simulink model "filecuaho"  (R2016b)
settings: Solver=VariableStepAuto  StartTime=0.0  StopTime=10.0  RelTol=1e-3
undefined symbols (not defined in the file): KACC_ACCT_CLR_NIDL_INIT, KACC_ACCUT_STATE_A, KACC_ACCUT_STATE_B, KACC_ACCUT_SW, KACC_ACTQSW, KACC_CLD, KACC_CLD_REQ_HYS, KACC_CLD_REQ_SW, KACC_COLPD, KACC_COMP_INRT, KACC_COMPTYPE_FIXED, KACC_COMPTYPE_VAR, KACC_CTTM_ACE, KACC_CTTM_ACON, KACC_CTTM_CRK, KACC_CTTM_FAN, KACC_CTTM_GRD, KACC_CTTM_IRS, KACC_CTTM_NAC, KACC_DIFFEVATEMPMAX, KACC_DIFFEVATEMPMIN, KACC_EVAT_ELSE, KACC_EVAT_ELSE_SW, KACC_EVATMPCUT_SW, KACC_EVATUPL_ELSE, KACC_EVATUPL_ELSE_SW, KACC_FANREQ_SW, KACC_FORCEDACON, KACC_HCAPS, KACC_HCAPS_HYS, KACC_HCCTTM, KACC_HCGRA, KACC_HCGRA_HYS, KACC_HCRGR, KACC_HCVS1, KACC_HCVS1_HYS, KACC_HCVS2, KACC_HCVS2_HYS, KACC_HEATUP_CE, KACC_HEATUP_CE_HYS, KACC_HEATUP_DRV2IDL, KACC_HEATUP_IDL2DRV, KACC_HEATUP_NE, KACC_HEATUP_NE_HYS, KACC_HIPS_ACOF, KACC_HIPS_ACON, KACC_LOPS_ACOF, KACC_LOPS_ACON, KACC_LYR3TR_ACHLD, KACC_NEW_RPM, KACC_OFDL_SW, KACC_OFDL_VCV, KACC_ONDL_SW, KACC_RECCP, KACC_RECCP_HYS, KACC_RECDLY, KACC_RECVS, KACC_S1_THWMAX, KACC_S1TM_THWULMT, KACC_SHLT_2CYL ... (+137)
libraries: lib2011b x727, SUBSYSTEM_LIB_CNV x30, SUBSYSTEM_LIB_ESC x2, SUBSYSTEM_LIB_AUX x1
(part 5 of 5)

== system filecuaho/acc_xaccuton/acc_accutreq/cal_cuttime ==
  note: 加速要求エアコンカットフラグ
  note: エアコンカット要求前にvcvcut要求があった場合は、
      | vcvcutを実行した時間だけエアコンカット維持時間をoffsetする
  xlacni : Inport
  xlacfs : Inport  Port=2
  xlacfs_iss : Inport  Port=3
  w_vcv_cut_time : Inport  Port=4
  xacct1 : Inport  Port=5
  xacct4 : Inport  Port=6
  xacuthil : Inport  Port=7
  xactempcut : Inport  Port=8
  MC_Add3 : lib2011b/Simulink Original/Math Operations/MC_Add  Inputs=+-  CollapseDim=1  SampleTime=-1  InputSameDT=on  OutMin=[]  OutMax=[]  OutDataTypeStr=single
  MC_Constant : lib2011b/Simulink Original/Sources/MC_Constant  Value=KACC_CTTM_NAC  datatype=Inherit: Inherit from 'Constant value'  SampleTime=inf  FramePeriod=inf  OutMin=[]  OutMax=[]  OutDataTypeStr=Inherit: Inherit from 'Constant value'
  MC_Constant1 : lib2011b/Simulink Original/Sources/MC_Constant  Value=KACC_CTTM_CRK  datatype=Inherit: Inherit from 'Constant value'  SampleTime=inf  FramePeriod=inf  OutMin=[]  OutMax=[]  OutDataTypeStr=Inherit: Inherit from 'Constant value'
  MC_Constant4 : lib2011b/Simulink Original/Sources/MC_Constant  Value=KACC_CTTM_IRS  datatype=Inherit: Inherit from 'Constant value'  SampleTime=inf  FramePeriod=inf  OutMin=[]  OutMax=[]  OutDataTypeStr=Inherit: Inherit from 'Constant value'
  MC_Constant5 : lib2011b/Simulink Original/Sources/MC_Constant  Value=KACC_CTTM_GRD  datatype=Inherit: Inherit from 'Constant value'  SampleTime=inf  FramePeriod=inf  OutMin=[]  OutMax=[]  OutDataTypeStr=Inherit: Inherit from 'Constant value'
  MC_Constant{6..9} (4 alike) : lib2011b/Simulink Original/Sources/MC_Constant  Value=0  datatype=single  SampleTime=inf  FramePeriod=inf  OutMin=[]  OutMax=[]  OutDataTypeStr=single
  MC_Edge2 : lib2011b/Mazda Library/Other/MC_Edge
  MC_LogicalOperator : lib2011b/Simulink Original/Logic and Bit Operations/MC_LogicalOperator  SelectedOperator=NOT  Inputs=2  SampleTime=-1  AllPortsSameDT=off  OutDataTypeStr=boolean
  MC_LogicalOperator1 : lib2011b/Simulink Original/Logic and Bit Operations/MC_LogicalOperator  SelectedOperator=OR  Inputs=3  SampleTime=-1  AllPortsSameDT=off  OutDataTypeStr=boolean
  MC_LogicalOperator3 : lib2011b/Simulink Original/Logic and Bit Operations/MC_LogicalOperator  SelectedOperator=OR  Inputs=4  SampleTime=-1  AllPortsSameDT=off  OutDataTypeStr=boolean
  MC_MinMax : lib2011b/Simulink Original/Math Operations/MC_MinMax  Function=max  Inputs=4  SampleTime=-1  InputSameDT=on  OutMin=[]  OutMax=[]
  MC_Switch{1,3..4,6} (4 alike) : lib2011b/Simulink Original/Signal Routing/MC_Switch  Criteria=u2 ~= 0  Threshold=0  SampleTime=-1  InputSameDT=on  OutMin=[]  OutMax=[]  AllowDiffInputSizes=off
  MC_UnitDelay1 : lib2011b/Simulink Original/Discrete/MC_UnitDelay  InitialCondition=0  InputProcessing=Inherited  SampleTime=-1  StateName=delay_yclcn_b20m9498
      settings: StateMustResolveToSignalObject=off  StateStorageClass=ExportedGlobal
  Switch5 : lib2011b/Simulink Original/Signal Routing/MC_Switch  Criteria=u2 ~= 0  Threshold=0  SampleTime=-1  InputSameDT=on  OutMin=[]  OutMax=[]  AllowDiffInputSizes=off
  xaccut_wicnt : Outport
  accut_reqtime : Outport  Port=2
  wires:
  MC_Constant/1 -> MC_Switch4/1
  MC_Constant1/1 -> MC_Switch1/1
  MC_Constant4/1 -> MC_Switch3/1
  [xlacfs] -> MC_Switch1/2
  xlacni/1 -> [xlacni]
  xlacfs/1 -> [xlacfs]
  xlacfs_iss/1 -> [xlacfs_iss]
  [xlacni] -> MC_Switch4/2
  [xlacfs_iss] -> MC_Switch3/2
  MC_MinMax/1 -> MC_Add3/1  "accut_reqtime_pre"
  [xlacni] -> MC_LogicalOperator1/1
  [xlacfs] -> MC_LogicalOperator1/2
  [xlacfs_iss] -> MC_LogicalOperator1/3
  MC_LogicalOperator1/1 -> xaccut_wicnt/1, MC_LogicalOperator/1  "xaccut_wicnt"
  MC_Constant5/1 -> MC_Switch6/1
  MC_Constant6/1 -> MC_Switch6/3
  MC_Constant8/1 -> MC_Switch1/3
  MC_Constant9/1 -> MC_Switch3/3
  MC_LogicalOperator/1 -> MC_Switch6/2
  MC_Constant7/1 -> MC_Switch4/3
  MC_Switch6/1 -> MC_MinMax/1
  MC_Switch4/1 -> MC_MinMax/2
  MC_Switch1/1 -> MC_MinMax/3
  MC_Switch3/1 -> MC_MinMax/4
  w_vcv_cut_time/1 -> [w_vcv_cut_time]  "w_vcv_cut_time"
  xacct1/1 -> [xacct1]
  xacct4/1 -> [xacct4]
  xacuthil/1 -> [xacuthil]
  xactempcut/1 -> [xactempcut]
  MC_Edge2/1 -> Switch5/2
  Switch5/1 -> MC_UnitDelay1/1, MC_Add3/2
  MC_UnitDelay1/1 -> Switch5/3
  [w_vcv_cut_time] -> Switch5/1
  MC_LogicalOperator3/1 -> MC_Edge2/1
  [xacct1] -> MC_LogicalOperator3/1
  [xacct4] -> MC_LogicalOperator3/2
  [xacuthil] -> MC_LogicalOperator3/3
  [xactempcut] -> MC_LogicalOperator3/4
  MC_Add3/1 -> accut_reqtime/1  "accut_reqtime"

== system filecuaho/acc_xaccuton/acc_accutreq/do_xacct1 ==
  xrload : Inport
  apsfil : Inport  Port=2
  gearp : Inport  Port=3
  w_tsmpl : Inport  Port=4
  Constant1 : lib2011b/Simulink Original/Sources/MC_Constant  Value=KSAVAC  datatype=Inherit: Inherit from 'Constant value'  SampleTime=inf  FramePeriod=inf  OutMin=[]  OutMax=[]  OutDataTypeStr=Inherit: Inherit from 'Constant value'
  Constant11 : lib2011b/Simulink Original/Sources/MC_Constant  Value=KSAVAC_HYS  datatype=Inherit: Inherit from 'Constant value'  SampleTime=inf  FramePeriod=inf  OutMin=[]  OutMax=[]  OutDataTypeStr=Inherit: Inherit from 'Constant value'
  LogicalOperator10 : lib2011b/Simulink Original/Logic and Bit Operations/MC_LogicalOperator  SelectedOperator=AND  Inputs=2  SampleTime=-1  AllPortsSameDT=off  OutDataTypeStr=boolean
  MC_Constant1 : lib2011b/Simulink Original/Sources/MC_Constant  Value=true  datatype=Inherit: Inherit from 'Constant value'  SampleTime=inf  FramePeriod=inf  OutMin=[]  OutMax=[]  OutDataTypeStr=Inherit: Inherit from 'Constant value'
  MC_Constant5 : lib2011b/Simulink Original/Sources/MC_Constant  Value=false  datatype=Inherit: Inherit from 'Constant value'  SampleTime=inf  FramePeriod=inf  OutMin=[]  OutMax=[]  OutDataTypeStr=Inherit: Inherit from 'Constant value'
  MC_Constant7 : lib2011b/Simulink Original/Sources/MC_Constant  Value=0  datatype=single  SampleTime=inf  FramePeriod=inf  OutMin=[]  OutMax=[]  OutDataTypeStr=single
  MC_DownCountTimer : lib2011b/Mazda Library/Timer/MC_DownCountTimer
      settings: AttributesFormatString=DownCountTimer
  MC_Edge : SUBSYSTEM_LIB_CNV/RiseEdge
      settings: AttributesFormatString=RISE
  MC_Hysteresis4 : SUBSYSTEM_LIB_CNV/TrueHys
      settings: AttributesFormatString=True
  MC_LogicalOperator : lib2011b/Simulink Original/Logic and Bit Operations/MC_LogicalOperator  SelectedOperator=NOT  Inputs=2  SampleTime=-1  AllPortsSameDT=off  OutDataTypeStr=boolean
  MC_RelationalOperator3 : lib2011b/Simulink Original/Logic and Bit Operations/MC_RelationalOperator  Operator=>  SampleTime=-1  InputSameDT=on  OutDataTypeStr=boolean
  MC_Table : lib2011b/Simulink Original/Lookup Tables/MC_Table_i  Label=TACC_TLACT  InputValues=TACC_TLACT_X  calsw_x=off  OutputValues=TACC_TLACT_Y  LsbValue=LSB_TACC_TLACT_Y  OffsetValue=OFFSET_TACC_TLACT_Y
      settings: AttributesFormatString=%<Label>\nX-axis %<calsw_x>
  xacct1 : Outport
  wires:
  apsfil/1 -> MC_Hysteresis4/1
  xrload/1 -> LogicalOperator10/1
  MC_Hysteresis4/1 -> LogicalOperator10/2  "xavact"
  Constant11/1 -> MC_Hysteresis4/3
  Constant1/1 -> MC_Hysteresis4/2
  MC_Constant5/1 -> MC_Edge/2
  LogicalOperator10/1 -> MC_Edge/1, MC_LogicalOperator/1
  MC_Constant1/1 -> MC_DownCountTimer/3
  MC_LogicalOperator/1 -> MC_DownCountTimer/1
  MC_Constant7/1 -> MC_RelationalOperator3/2
  MC_DownCountTimer/1 -> MC_RelationalOperator3/1  "tacct1"
  MC_RelationalOperator3/1 -> xacct1/1  "xacct1"
  w_tsmpl/1 -> MC_DownCountTimer/5
  gearp/1 -> MC_Table/1
  MC_Table/1 -> MC_DownCountTimer/4
  MC_Edge/1 -> MC_DownCountTimer/2  "xacct1_req"

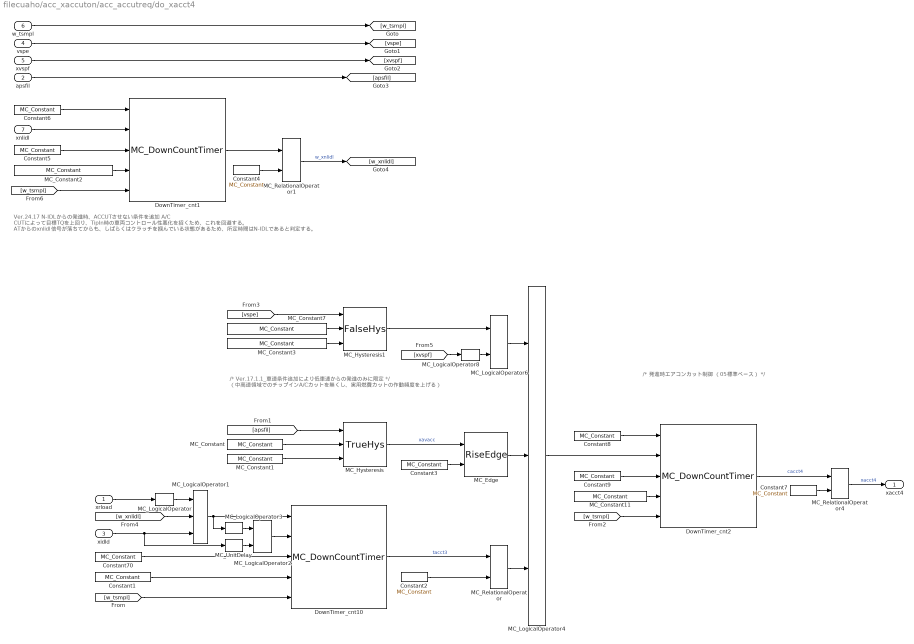
== system filecuaho/acc_xaccuton/acc_accutreq/do_xacct4 ==
  note: /* 発進時エアコンカット制御 （05標準ベース） */
  note: /* Ver.17.1.1_車速条件追加により低車速からの発進のみに限定 */
      |
      | （中高速領域でのチップインA/Cカットを無くし、実用燃費カットの作動頻度を上げる）
  note: Ver.24.17 N-IDLからの発進時、ACCUTさせない条件を追加
      | A/C CUTによって目標TQを上回り、TipIn時の車両コントロール性悪化を招くため、これを回避する。
      | ATからのxnlidl信号が落ちてからも、しばらくはクラッチを掴んでいる状態があるため、所定時間はN-IDLであると判定する。
  xrload : Inport
  apsfil : Inport  Port=2
  xidld : Inport  Port=3
  vspe : Inport  Port=4
  xvspf : Inport  Port=5
  w_tsmpl : Inport  Port=6
  xnlidl : Inport  Port=7
  Constant1 : lib2011b/Simulink Original/Sources/MC_Constant  Value=KLACT3  datatype=Inherit: Inherit from 'Constant value'  SampleTime=inf  FramePeriod=inf  OutMin=[]  OutMax=[]  OutDataTypeStr=Inherit: Inherit from 'Constant value'
  Constant2 : lib2011b/Simulink Original/Sources/MC_Constant  Value=0  datatype=single  SampleTime=inf  FramePeriod=inf  OutMin=[]  OutMax=[]  OutDataTypeStr=single
  Constant3 : lib2011b/Simulink Original/Sources/MC_Constant  Value=false  datatype=Inherit: Inherit from 'Constant value'  SampleTime=inf  FramePeriod=inf  OutMin=[]  OutMax=[]  OutDataTypeStr=Inherit: Inherit from 'Constant value'
  Constant4 : lib2011b/Simulink Original/Sources/MC_Constant  Value=0  datatype=single  SampleTime=inf  FramePeriod=inf  OutMin=[]  OutMax=[]  OutDataTypeStr=single
  Constant5 : lib2011b/Simulink Original/Sources/MC_Constant  Value=true  datatype=Inherit: Inherit from 'Constant value'  SampleTime=inf  FramePeriod=inf  OutMin=[]  OutMax=[]  OutDataTypeStr=Inherit: Inherit from 'Constant value'
  Constant6 : lib2011b/Simulink Original/Sources/MC_Constant  Value=false  datatype=Inherit: Inherit from 'Constant value'  SampleTime=inf  FramePeriod=inf  OutMin=[]  OutMax=[]  OutDataTypeStr=Inherit: Inherit from 'Constant value'
  Constant7 : lib2011b/Simulink Original/Sources/MC_Constant  Value=0  datatype=single  SampleTime=inf  FramePeriod=inf  OutMin=[]  OutMax=[]  OutDataTypeStr=single
  Constant70 : lib2011b/Simulink Original/Sources/MC_Constant  Value=true  datatype=Inherit: Inherit from 'Constant value'  SampleTime=inf  FramePeriod=inf  OutMin=[]  OutMax=[]  OutDataTypeStr=Inherit: Inherit from 'Constant value'
  Constant8 : lib2011b/Simulink Original/Sources/MC_Constant  Value=false  datatype=Inherit: Inherit from 'Constant value'  SampleTime=inf  FramePeriod=inf  OutMin=[]  OutMax=[]  OutDataTypeStr=Inherit: Inherit from 'Constant value'
  Constant9 : lib2011b/Simulink Original/Sources/MC_Constant  Value=true  datatype=Inherit: Inherit from 'Constant value'  SampleTime=inf  FramePeriod=inf  OutMin=[]  OutMax=[]  OutDataTypeStr=Inherit: Inherit from 'Constant value'
  DownTimer_cnt1 : lib2011b/Mazda Library/Timer/MC_DownCountTimer
      settings: AttributesFormatString=DownCountTimer
  DownTimer_cnt10 : lib2011b/Mazda Library/Timer/MC_DownCountTimer
      settings: AttributesFormatString=DownCountTimer
  DownTimer_cnt2 : lib2011b/Mazda Library/Timer/MC_DownCountTimer
      settings: AttributesFormatString=DownCountTimer
  MC_Constant : lib2011b/Simulink Original/Sources/MC_Constant  Value=KSAVCC  datatype=Inherit: Inherit from 'Constant value'  SampleTime=inf  FramePeriod=inf  OutMin=[]  OutMax=[]  OutDataTypeStr=Inherit: Inherit from 'Constant value'
  MC_Constant1 : lib2011b/Simulink Original/Sources/MC_Constant  Value=KSAVCC_HYS  datatype=Inherit: Inherit from 'Constant value'  SampleTime=inf  FramePeriod=inf  OutMin=[]  OutMax=[]  OutDataTypeStr=Inherit: Inherit from 'Constant value'
  MC_Constant11 : lib2011b/Simulink Original/Sources/MC_Constant  Value=KACC_CTTM_ACE  datatype=Inherit: Inherit from 'Constant value'  SampleTime=inf  FramePeriod=inf  OutMin=[]  OutMax=[]  OutDataTypeStr=Inherit: Inherit from 'Constant value'
  MC_Constant2 : lib2011b/Simulink Original/Sources/MC_Constant  Value=KACC_ACCT_CLR_NIDL_INIT  datatype=Inherit: Inherit from 'Constant value'  SampleTime=inf  FramePeriod=inf  OutMin=[]  OutMax=[]  OutDataTypeStr=Inherit: Inherit from 'Constant value'
  MC_Constant3 : lib2011b/Simulink Original/Sources/MC_Constant  Value=KACC_START_VSP_HYS  datatype=Inherit: Inherit from 'Constant value'  SampleTime=inf  FramePeriod=inf  OutMin=[]  OutMax=[]  OutDataTypeStr=Inherit: Inherit from 'Constant value'
  MC_Constant7 : lib2011b/Simulink Original/Sources/MC_Constant  Value=KACC_START_VSP  datatype=Inherit: Inherit from 'Constant value'  SampleTime=inf  FramePeriod=inf  OutMin=[]  OutMax=[]  OutDataTypeStr=Inherit: Inherit from 'Constant value'
  MC_Edge : SUBSYSTEM_LIB_CNV/RiseEdge
      settings: AttributesFormatString=RISE
  MC_Hysteresis : SUBSYSTEM_LIB_CNV/TrueHys
      settings: AttributesFormatString=True
  MC_Hysteresis1 : SUBSYSTEM_LIB_CNV/FalseHys
      settings: AttributesFormatString=False
  MC_LogicalOperator : lib2011b/Simulink Original/Logic and Bit Operations/MC_LogicalOperator  SelectedOperator=NOT  Inputs=2  SampleTime=-1  AllPortsSameDT=off  OutDataTypeStr=boolean
  MC_LogicalOperator1 : lib2011b/Simulink Original/Logic and Bit Operations/MC_LogicalOperator  SelectedOperator=OR  Inputs=3  SampleTime=-1  AllPortsSameDT=off  OutDataTypeStr=boolean
  MC_LogicalOperator2 : lib2011b/Simulink Original/Logic and Bit Operations/MC_LogicalOperator  SelectedOperator=AND  Inputs=2  SampleTime=-1  AllPortsSameDT=off  OutDataTypeStr=boolean
  MC_LogicalOperator3 : lib2011b/Simulink Original/Logic and Bit Operations/MC_LogicalOperator  SelectedOperator=NOT  Inputs=2  SampleTime=-1  AllPortsSameDT=off  OutDataTypeStr=boolean
  MC_LogicalOperator4 : lib2011b/Simulink Original/Logic and Bit Operations/MC_LogicalOperator  SelectedOperator=AND  Inputs=3  SampleTime=-1  AllPortsSameDT=off  OutDataTypeStr=boolean
  MC_LogicalOperator6 : lib2011b/Simulink Original/Logic and Bit Operations/MC_LogicalOperator  SelectedOperator=AND  Inputs=2  SampleTime=-1  AllPortsSameDT=off  OutDataTypeStr=boolean
  MC_LogicalOperator8 : lib2011b/Simulink Original/Logic and Bit Operations/MC_LogicalOperator  SelectedOperator=NOT  Inputs=2  SampleTime=-1  AllPortsSameDT=off  OutDataTypeStr=boolean
  MC_RelationalOperator : lib2011b/Simulink Original/Logic and Bit Operations/MC_RelationalOperator  Operator=>  SampleTime=-1  InputSameDT=on  OutDataTypeStr=boolean
  MC_RelationalOperator1 : lib2011b/Simulink Original/Logic and Bit Operations/MC_RelationalOperator  Operator=>  SampleTime=-1  InputSameDT=on  OutDataTypeStr=boolean
  MC_RelationalOperator4 : lib2011b/Simulink Original/Logic and Bit Operations/MC_RelationalOperator  Operator=>  SampleTime=-1  InputSameDT=on  OutDataTypeStr=boolean
  MC_UnitDelay : lib2011b/Simulink Original/Discrete/MC_UnitDelay  InitialCondition=0  InputProcessing=Inherited  SampleTime=-1  StateName=delay_yclcn_b20m9499
      settings: StateMustResolveToSignalObject=off  StateStorageClass=ExportedGlobal
  xacct4 : Outport
  wires:
  MC_Constant1/1 -> MC_Hysteresis/3
  MC_Constant/1 -> MC_Hysteresis/2
  MC_LogicalOperator2/1 -> DownTimer_cnt10/2
  MC_UnitDelay/1 -> MC_LogicalOperator2/2
  MC_LogicalOperator3/1 -> MC_LogicalOperator2/1
  xidld/1 -> MC_UnitDelay/1, MC_LogicalOperator1/3
  MC_LogicalOperator/1 -> MC_LogicalOperator1/1
  MC_LogicalOperator1/1 -> DownTimer_cnt10/1, MC_LogicalOperator3/1
  xrload/1 -> MC_LogicalOperator/1
  Constant1/1 -> DownTimer_cnt10/4
  Constant70/1 -> DownTimer_cnt10/3
  Constant3/1 -> MC_Edge/2
  Constant2/1 -> MC_RelationalOperator/2
  DownTimer_cnt10/1 -> MC_RelationalOperator/1  "tacct3"
  MC_Hysteresis/1 -> MC_Edge/1  "xavacc"
  w_tsmpl/1 -> [w_tsmpl]
  [w_tsmpl] -> DownTimer_cnt10/5
  MC_RelationalOperator/1 -> MC_LogicalOperator4/3
  MC_LogicalOperator4/1 -> DownTimer_cnt2/2
  [w_tsmpl] -> DownTimer_cnt2/5
  Constant8/1 -> DownTimer_cnt2/1
  Constant9/1 -> DownTimer_cnt2/3
  MC_RelationalOperator4/1 -> xacct4/1  "xacct4"
  DownTimer_cnt2/1 -> MC_RelationalOperator4/1  "cacct4"
  vspe/1 -> [vspe]
  xvspf/1 -> [xvspf]
  [xvspf] -> MC_LogicalOperator8/1
  MC_Constant11/1 -> DownTimer_cnt2/4
  Constant7/1 -> MC_RelationalOperator4/2
  MC_Edge/1 -> MC_LogicalOperator4/2
  MC_LogicalOperator6/1 -> MC_LogicalOperator4/1
  MC_LogicalOperator8/1 -> MC_LogicalOperator6/2
  MC_Hysteresis1/1 -> MC_LogicalOperator6/1
  [vspe] -> MC_Hysteresis1/1
  MC_Constant7/1 -> MC_Hysteresis1/2
  MC_Constant3/1 -> MC_Hysteresis1/3
  apsfil/1 -> [apsfil]
  [apsfil] -> MC_Hysteresis/1
  xnlidl/1 -> DownTimer_cnt1/2
  [w_xnlidl] -> MC_LogicalOperator1/2
  Constant4/1 -> MC_RelationalOperator1/2
  DownTimer_cnt1/1 -> MC_RelationalOperator1/1
  MC_RelationalOperator1/1 -> [w_xnlidl]  "w_xnlidl"
  Constant5/1 -> DownTimer_cnt1/3
  Constant6/1 -> DownTimer_cnt1/1
  [w_tsmpl] -> DownTimer_cnt1/5
  MC_Constant2/1 -> DownTimer_cnt1/4

== system filecuaho/acc_xaccuton/acc_accutreq/do_xacflostcut ==
  xcol : Inport
  evatemp : Inport  Port=2
  Constant14 : lib2011b/Simulink Original/Sources/MC_Constant  Value=KACC_VCD_EVATMP_HYS  datatype=Inherit: Inherit from 'Constant value'  SampleTime=inf  FramePeriod=inf  OutMin=[]  OutMax=[]  OutDataTypeStr=Inherit: Inherit from 'Constant value'
  Constant5 : lib2011b/Simulink Original/Sources/MC_Constant  Value=KACC_VCD_EVATMP  datatype=Inherit: Inherit from 'Constant value'  SampleTime=inf  FramePeriod=inf  OutMin=[]  OutMax=[]  OutDataTypeStr=Inherit: Inherit from 'Constant value'
  MC_Add : lib2011b/Simulink Original/Math Operations/MC_Add  Inputs=++  CollapseDim=1  SampleTime=-1  OutMin=[]  OutMax=[]  OutDataTypeStr=single
  MC_Hysteresis : lib2011b/Mazda Library/Other/MC_Hysteresis  outtype=False
      settings: AttributesFormatString=%<outtype>
  MC_LogicalOperator4 : lib2011b/Simulink Original/Logic and Bit Operations/MC_LogicalOperator  SelectedOperator=AND  Inputs=2  SampleTime=-1  AllPortsSameDT=off  OutDataTypeStr=boolean
  MC_LogicalOperator5 : lib2011b/Simulink Original/Logic and Bit Operations/MC_LogicalOperator  SelectedOperator=NOT  Inputs=2  SampleTime=-1  AllPortsSameDT=off  OutDataTypeStr=boolean
  xacflostcut : Outport
  wires:
  xcol/1 -> MC_LogicalOperator5/1
  MC_LogicalOperator5/1 -> MC_LogicalOperator4/1
  Constant5/1 -> MC_Hysteresis/3, MC_Add/2
  Constant14/1 -> MC_Add/1
  MC_Add/1 -> MC_Hysteresis/2
  evatemp/1 -> MC_Hysteresis/1
  MC_Hysteresis/1 -> MC_LogicalOperator4/2
  MC_LogicalOperator4/1 -> xacflostcut/1  "xacflostcut"

== system filecuaho/acc_xaccuton/acc_accutreq/do_xacfrpm ==
  ne : Inport
  xclcn : Inport  Port=2
  xaltcalflg : Inport  Port=3
  MC_Add : lib2011b/Simulink Original/Math Operations/MC_Add  Inputs=-+  CollapseDim=1  SampleTime=-1  InputSameDT=on  OutMin=[]  OutMax=[]  OutDataTypeStr=single
  MC_BackUp : lib2011b/Mazda Library/ControlFunction/MC_BackUp  x0=KACC_CNTDWN
      settings: AttributesFormatString=RESET = %<x0>
  MC_Constant : lib2011b/Simulink Original/Sources/MC_Constant  Value=KACC_NEW_RPM  datatype=Inherit: Inherit from 'Constant value'  SampleTime=inf  FramePeriod=inf  OutMin=[]  OutMax=[]  OutDataTypeStr=Inherit: Inherit from 'Constant value'
  MC_Constant1 : lib2011b/Simulink Original/Sources/MC_Constant  Value=0  datatype=single  SampleTime=inf  FramePeriod=inf  OutMin=[]  OutMax=[]  OutDataTypeStr=single
  MC_Constant2 : lib2011b/Simulink Original/Sources/MC_Constant  Value=1  datatype=single  SampleTime=inf  FramePeriod=inf  OutMin=[]  OutMax=[]  OutDataTypeStr=single
  MC_Constant3 : lib2011b/Simulink Original/Sources/MC_Constant  Value=false  datatype=Inherit: Inherit from 'Constant value'  SampleTime=inf  FramePeriod=inf  OutMin=[]  OutMax=[]  OutDataTypeStr=Inherit: Inherit from 'Constant value'
  MC_Edge : SUBSYSTEM_LIB_CNV/FallEdge
      settings: AttributesFormatString=FALL
  MC_LogicalOperator : lib2011b/Simulink Original/Logic and Bit Operations/MC_LogicalOperator  SelectedOperator=AND  Inputs=3  SampleTime=-1  AllPortsSameDT=off  OutDataTypeStr=boolean
  MC_RelationalOperator : lib2011b/Simulink Original/Logic and Bit Operations/MC_RelationalOperator  Operator=>=  SampleTime=-1  InputSameDT=on  OutDataTypeStr=boolean
  MC_RelationalOperator1 : lib2011b/Simulink Original/Logic and Bit Operations/MC_RelationalOperator  Operator=>  SampleTime=-1  InputSameDT=on  OutDataTypeStr=boolean
  MC_Saturation : lib2011b/Simulink Original/Discontinuities/MC_Saturation  msk_max=KACC_CNTDWN  msk_min=0
      settings: AttributesFormatString=MAX = %<msk_max>\nMIN = %<msk_min>
  MC_Switch : lib2011b/Simulink Original/Signal Routing/MC_Switch  Criteria=u2 ~= 0  Threshold=0  SampleTime=-1  InputSameDT=on  OutMin=[]  OutMax=[]  AllowDiffInputSizes=off
  xacfrpm : Outport
  wires:
  MC_LogicalOperator/1 -> xacfrpm/1  "xacfrpm"
  MC_Constant/1 -> MC_RelationalOperator/2
  ne/1 -> MC_RelationalOperator/1
  xclcn/1 -> MC_Edge/1
  MC_Constant1/1 -> MC_RelationalOperator1/2
  MC_Switch/1 -> MC_Saturation/1
  MC_Saturation/1 -> MC_RelationalOperator1/1, MC_BackUp/1  "cacfrpm_cntdwn"
  MC_BackUp/1 -> MC_Switch/3, MC_Add/2
  MC_Add/1 -> MC_Switch/1
  MC_Constant2/1 -> MC_Add/1
  MC_Constant3/1 -> MC_Edge/2
  MC_Edge/1 -> MC_Switch/2
  xaltcalflg/1 -> MC_LogicalOperator/1
  MC_RelationalOperator/1 -> MC_LogicalOperator/2
  MC_RelationalOperator1/1 -> MC_LogicalOperator/3

== system filecuaho/acc_xaccuton/acc_accutreq/do_xacpcut ==
  colp : Inport
  w_tsmpl : Inport  Port=2
  MC_Constant2 : lib2011b/Simulink Original/Sources/MC_Constant  Value=KSCOLP  datatype=Inherit: Inherit from 'Constant value'  SampleTime=inf  FramePeriod=inf  OutMin=[]  OutMax=[]  OutDataTypeStr=Inherit: Inherit from 'Constant value'
  MC_Constant3 : lib2011b/Simulink Original/Sources/MC_Constant  Value=KSCOLPHY  datatype=Inherit: Inherit from 'Constant value'  SampleTime=inf  FramePeriod=inf  OutMin=[]  OutMax=[]  OutDataTypeStr=Inherit: Inherit from 'Constant value'
  MC_Hysteresis3 : SUBSYSTEM_LIB_CNV/TrueHys
      settings: AttributesFormatString=True
  MC_LogicalOperator : lib2011b/Simulink Original/Logic and Bit Operations/MC_LogicalOperator  SelectedOperator=OR  Inputs=2  SampleTime=-1  AllPortsSameDT=off  OutDataTypeStr=boolean
  xcolphi : Subsystem
  xcolplo : Subsystem
  xacpcut : Outport
  xcolp : Outport  Port=2
  wires:
  xcolplo/1(xcolplo) -> MC_LogicalOperator/2
  xcolphi/1(xcolphi) -> MC_LogicalOperator/1
  w_tsmpl/1 -> xcolplo/2(w_tsmpl)
  MC_Constant2/1 -> MC_Hysteresis3/2
  MC_Constant3/1 -> MC_Hysteresis3/3
  colp/1 -> xcolplo/1(colp), MC_Hysteresis3/1, xcolphi/1(colp)
  MC_LogicalOperator/1 -> xacpcut/1  "xacpcut"
  MC_Hysteresis3/1 -> xcolp/1  "xcolp"

== system filecuaho/acc_xaccuton/acc_accutreq/do_xactempcut ==
  evatemp_uplmt : Inport
  evatemp : Inport  Port=2
  apsfil : Inport  Port=3
  MC_Add : lib2011b/Simulink Original/Math Operations/MC_Add  Inputs=+-  CollapseDim=1  SampleTime=-1  InputSameDT=on  OutMin=[]  OutMax=[]  OutDataTypeStr=single
  MC_Constant : lib2011b/Simulink Original/Sources/MC_Constant  Value=KACC_DIFFEVATEMPMIN  datatype=Inherit: Inherit from 'Constant value'  SampleTime=inf  FramePeriod=inf  OutMin=[]  OutMax=[]  OutDataTypeStr=Inherit: Inherit from 'Constant value'
  MC_Constant1 : lib2011b/Simulink Original/Sources/MC_Constant  Value=KACC_DIFFEVATEMPMAX  datatype=Inherit: Inherit from 'Constant value'  SampleTime=inf  FramePeriod=inf  OutMin=[]  OutMax=[]  OutDataTypeStr=Inherit: Inherit from 'Constant value'
  MC_Constant2 : lib2011b/Simulink Original/Sources/MC_Constant  Value=0  datatype=single  SampleTime=inf  FramePeriod=inf  OutMin=[]  OutMax=[]  OutDataTypeStr=single
  MC_Edge2 : lib2011b/Mazda Library/Other/MC_Edge
  MC_LogicalOperator4 : lib2011b/Simulink Original/Logic and Bit Operations/MC_LogicalOperator  SelectedOperator=AND  Inputs=2  SampleTime=-1  AllPortsSameDT=off  OutDataTypeStr=boolean
  MC_RelationalOperator1 : lib2011b/Simulink Original/Logic and Bit Operations/MC_RelationalOperator  Operator=<=  SampleTime=-1  InputSameDT=on  OutDataTypeStr=boolean
  MC_RelationalOperator2 : lib2011b/Simulink Original/Logic and Bit Operations/MC_RelationalOperator  Operator=>  SampleTime=-1  InputSameDT=on  OutDataTypeStr=boolean
  MC_RelationalOperator4 : lib2011b/Simulink Original/Logic and Bit Operations/MC_RelationalOperator  Operator=>=  SampleTime=-1  InputSameDT=on  OutDataTypeStr=boolean
  MC_SetFlag1 : lib2011b/Mazda Library/Other/MC_SetFlag
      settings: AttributesFormatString=SetFlag
  xactempcut : Outport
  wires:
  MC_LogicalOperator4/1 -> MC_SetFlag1/2
  MC_SetFlag1/1 -> xactempcut/1  "xactempcut"
  MC_Constant/1 -> MC_RelationalOperator1/2
  MC_RelationalOperator1/1 -> MC_SetFlag1/1
  MC_Constant1/1 -> MC_RelationalOperator4/2
  evatemp_uplmt/1 -> MC_Add/1
  evatemp/1 -> MC_Add/2
  MC_Add/1 -> MC_RelationalOperator4/1, MC_RelationalOperator1/1
  MC_RelationalOperator4/1 -> MC_LogicalOperator4/1
  MC_Edge2/1 -> MC_LogicalOperator4/2
  MC_RelationalOperator2/1 -> MC_Edge2/1
  apsfil/1 -> MC_RelationalOperator2/1
  MC_Constant2/1 -> MC_RelationalOperator2/2

== system filecuaho/acc_xaccuton/acc_accutreq/do_xacuthil ==
  note: ギヤ比（FGRを除く）
  note: /* grade（Gセンサから演算） */
      |
      | 車速微分と、ABS/DSCのGセンサ値から登降坂勾配を推定
      |
      | （登坂時＋、降坂時－）
  note: アクセル開度
  note: 車速
  note: /* 登坂時エアコンカット（低勾配側） */
      |
      | J68C ZYVへの織り込み仕様をスライド。
      |
      | "rgearが1速相当 && apsfil所定以上 && vspe所定以下"で7秒間エアコンカット実行。
      |
      | ただし、"apsfil所定以下 || vspe所定以上"でエアコン即復帰。
  note: /* 登坂時エアコンカット（高勾配側） */
      |
      | Ver.15.4.1で新規追加。
      |
      | "rgearが1速相当 && apsfil所定以上 && vspe所定以下"でエアコンカット実行。
      |
      | ただし、"apsfil所定以下 || vspe所定以上"でエアコン復帰。
      |
      | ※高勾配が長い時間続く場合、従来の登坂時カットではアクセルを踏み直す必要がある。
      | また、高勾配のエアコンカット状態でも車速が一定以上出ないため、車速条件を低勾配側とは別に設定する必要あり。
  vspe : Inport
  apsfil : Inport  Port=2
  rgear : Inport  Port=3
  grade : Inport  Port=4
  w_tsmpl : Inport  Port=5
  MC_Constant : lib2011b/Simulink Original/Sources/MC_Constant  Value=KACC_HCVS1  datatype=Inherit: Inherit from 'Constant value'  SampleTime=inf  FramePeriod=inf  OutMin=[]  OutMax=[]  OutDataTypeStr=Inherit: Inherit from 'Constant value'
  MC_Constant1 : lib2011b/Simulink Original/Sources/MC_Constant  Value=KACC_HCAPS  datatype=Inherit: Inherit from 'Constant value'  SampleTime=inf  FramePeriod=inf  OutMin=[]  OutMax=[]  OutDataTypeStr=Inherit: Inherit from 'Constant value'
  MC_Constant10 : lib2011b/Simulink Original/Sources/MC_Constant  Value=KACC_HCAPS_HYS  datatype=Inherit: Inherit from 'Constant value'  SampleTime=inf  FramePeriod=inf  OutMin=[]  OutMax=[]  OutDataTypeStr=Inherit: Inherit from 'Constant value'
  MC_Constant11 : lib2011b/Simulink Original/Sources/MC_Constant  Value=KACC_HCVS2  datatype=Inherit: Inherit from 'Constant value'  SampleTime=inf  FramePeriod=inf  OutMin=[]  OutMax=[]  OutDataTypeStr=Inherit: Inherit from 'Constant value'
  MC_Constant12 : lib2011b/Simulink Original/Sources/MC_Constant  Value=KACC_HCVS2_HYS  datatype=Inherit: Inherit from 'Constant value'  SampleTime=inf  FramePeriod=inf  OutMin=[]  OutMax=[]  OutDataTypeStr=Inherit: Inherit from 'Constant value'
  MC_Constant2 : lib2011b/Simulink Original/Sources/MC_Constant  Value=KACC_HCRGR  datatype=Inherit: Inherit from 'Constant value'  SampleTime=inf  FramePeriod=inf  OutMin=[]  OutMax=[]  OutDataTypeStr=Inherit: Inherit from 'Constant value'
  MC_Constant3 : lib2011b/Simulink Original/Sources/MC_Constant  Value=KACC_HCVS1_HYS  datatype=Inherit: Inherit from 'Constant value'  SampleTime=inf  FramePeriod=inf  OutMin=[]  OutMax=[]  OutDataTypeStr=Inherit: Inherit from 'Constant value'
  MC_Constant4 : lib2011b/Simulink Original/Sources/MC_Constant  Value=false  datatype=Inherit: Inherit from 'Constant value'  SampleTime=inf  FramePeriod=inf  OutMin=[]  OutMax=[]  OutDataTypeStr=Inherit: Inherit from 'Constant value'
  MC_Constant5 : lib2011b/Simulink Original/Sources/MC_Constant  Value=KACC_HCGRA  datatype=Inherit: Inherit from 'Constant value'  SampleTime=inf  FramePeriod=inf  OutMin=[]  OutMax=[]  OutDataTypeStr=Inherit: Inherit from 'Constant value'
  MC_Constant6 : lib2011b/Simulink Original/Sources/MC_Constant  Value=true  datatype=Inherit: Inherit from 'Constant value'  SampleTime=inf  FramePeriod=inf  OutMin=[]  OutMax=[]  OutDataTypeStr=Inherit: Inherit from 'Constant value'
  MC_Constant7 : lib2011b/Simulink Original/Sources/MC_Constant  Value=0  datatype=single  SampleTime=inf  FramePeriod=inf  OutMin=[]  OutMax=[]  OutDataTypeStr=single
  MC_Constant8 : lib2011b/Simulink Original/Sources/MC_Constant  Value=KACC_HCGRA_HYS  datatype=Inherit: Inherit from 'Constant value'  SampleTime=inf  FramePeriod=inf  OutMin=[]  OutMax=[]  OutDataTypeStr=Inherit: Inherit from 'Constant value'
  MC_Constant9 : lib2011b/Simulink Original/Sources/MC_Constant  Value=KACC_HCCTTM  datatype=Inherit: Inherit from 'Constant value'  SampleTime=inf  FramePeriod=inf  OutMin=[]  OutMax=[]  OutDataTypeStr=Inherit: Inherit from 'Constant value'
  MC_DownCountTimer : lib2011b/Mazda Library/Timer/MC_DownCountTimer
      settings: AttributesFormatString=DownCountTimer
  MC_Edge : SUBSYSTEM_LIB_CNV/RiseEdge
      settings: AttributesFormatString=RISE
  MC_Hysteresis{,1..3} (4 alike) : SUBSYSTEM_LIB_CNV/TrueHys
      settings: AttributesFormatString=True
  MC_LogicalOperator : lib2011b/Simulink Original/Logic and Bit Operations/MC_LogicalOperator  SelectedOperator=AND  Inputs=2  SampleTime=-1  AllPortsSameDT=off  OutDataTypeStr=boolean
  MC_LogicalOperator1 : lib2011b/Simulink Original/Logic and Bit Operations/MC_LogicalOperator  SelectedOperator=NOT  Inputs=2  SampleTime=-1  AllPortsSameDT=off  OutDataTypeStr=boolean
  MC_LogicalOperator2 : lib2011b/Simulink Original/Logic and Bit Operations/MC_LogicalOperator  SelectedOperator=OR  Inputs=2  SampleTime=-1  AllPortsSameDT=off  OutDataTypeStr=boolean
  MC_LogicalOperator3 : lib2011b/Simulink Original/Logic and Bit Operations/MC_LogicalOperator  SelectedOperator=NOT  Inputs=2  SampleTime=-1  AllPortsSameDT=off  OutDataTypeStr=boolean
  MC_LogicalOperator4 : lib2011b/Simulink Original/Logic and Bit Operations/MC_LogicalOperator  SelectedOperator=OR  Inputs=2  SampleTime=-1  AllPortsSameDT=off  OutDataTypeStr=boolean
  MC_LogicalOperator5 : lib2011b/Simulink Original/Logic and Bit Operations/MC_LogicalOperator  SelectedOperator=NOT  Inputs=2  SampleTime=-1  AllPortsSameDT=off  OutDataTypeStr=boolean
  MC_RelationalOperator2 : lib2011b/Simulink Original/Logic and Bit Operations/MC_RelationalOperator  Operator=>  SampleTime=-1  InputSameDT=on  OutDataTypeStr=boolean
  MC_RelationalOperator3 : lib2011b/Simulink Original/Logic and Bit Operations/MC_RelationalOperator  Operator=>  SampleTime=-1  InputSameDT=on  OutDataTypeStr=boolean
  MC_SetFlag : lib2011b/Mazda Library/Other/MC_SetFlag
      settings: AttributesFormatString=SetFlag
  MC_SetFlag1 : lib2011b/Mazda Library/Other/MC_SetFlag
      settings: AttributesFormatString=SetFlag
  MC_Switch : lib2011b/Simulink Original/Signal Routing/MC_Switch  Criteria=u2 ~= 0  Threshold=0  SampleTime=-1  InputSameDT=on  OutMin=[]  OutMax=[]  AllowDiffInputSizes=off
  xacuthil : Outport
  wires:
  rgear/1 -> MC_RelationalOperator2/1
  MC_Constant2/1 -> MC_RelationalOperator2/2
  MC_Constant/1 -> MC_Hysteresis/2
  MC_Constant3/1 -> MC_Hysteresis/3
  w_tsmpl/1 -> MC_DownCountTimer/5
  MC_Constant6/1 -> MC_DownCountTimer/3
  MC_DownCountTimer/1 -> MC_RelationalOperator3/1  "ctohan_lo"
  MC_Constant7/1 -> MC_RelationalOperator3/2
  MC_RelationalOperator2/1 -> MC_LogicalOperator/2
  MC_LogicalOperator1/1 -> MC_DownCountTimer/1
  MC_Edge/1 -> MC_DownCountTimer/2
  MC_Constant4/1 -> MC_Edge/2
  MC_SetFlag/1 -> MC_Edge/1, MC_LogicalOperator1/1  "xtohan_lo_cut"
  MC_LogicalOperator2/1 -> MC_SetFlag/1
  MC_Hysteresis/1 -> MC_LogicalOperator2/1
  grade/1 -> MC_Hysteresis1/1
  MC_Constant5/1 -> MC_Hysteresis1/2
  MC_Constant8/1 -> MC_Hysteresis1/3
  vspe/1 -> MC_Hysteresis/1, MC_Hysteresis2/1
  MC_RelationalOperator3/1 -> MC_Switch/3  "xtohan_lo"
  MC_Switch/1 -> xacuthil/1  "xacuthil"
  MC_Hysteresis1/1 -> MC_Switch/2
  MC_Constant12/1 -> MC_Hysteresis2/3
  MC_Hysteresis2/1 -> MC_LogicalOperator4/1
  MC_Constant11/1 -> MC_Hysteresis2/2
  MC_LogicalOperator4/1 -> MC_SetFlag1/1
  MC_SetFlag1/1 -> MC_Switch/1  "xtohan_hi"
  MC_Constant9/1 -> MC_DownCountTimer/4
  apsfil/1 -> MC_Hysteresis3/1
  MC_Constant1/1 -> MC_Hysteresis3/2
  MC_Constant10/1 -> MC_Hysteresis3/3
  MC_Hysteresis3/1 -> MC_LogicalOperator/1, MC_LogicalOperator5/1, MC_LogicalOperator3/1
  MC_LogicalOperator3/1 -> MC_LogicalOperator2/2
  MC_LogicalOperator5/1 -> MC_LogicalOperator4/2
  MC_LogicalOperator/1 -> MC_SetFlag1/2, MC_SetFlag/2

== system filecuaho/acc_xaccuton/acc_accutreq/do_xis_colof ==
  note: Ver24.13.1_追加
      | 有車速IS対応のため、iss_stateを見てIS条件ACカットフラグを成立させる。
  vspe : Inport
  xstbymd_iss : Inport  Port=2
  xismd_iss : Inport  Port=3
  xirmd_iss : Inport  Port=4
  iss_state : Inport  Port=5
  MC_Constant : lib2011b/Simulink Original/Sources/MC_Constant  Value=KCOLOFVSP  datatype=Inherit: Inherit from 'Constant value'  SampleTime=inf  FramePeriod=inf  OutMin=[]  OutMax=[]  OutDataTypeStr=Inherit: Inherit from 'Constant value'
  MC_Constant1 : lib2011b/Simulink Original/Sources/MC_Constant  Value=KACC_ACCUT_STATE_A  datatype=Inherit: Inherit from 'Constant value'  SampleTime=inf  FramePeriod=inf  OutMin=[]  OutMax=[]  OutDataTypeStr=Inherit: Inherit from 'Constant value'
  MC_Constant2 : lib2011b/Simulink Original/Sources/MC_Constant  Value=KACC_ACCUT_STATE_B  datatype=Inherit: Inherit from 'Constant value'  SampleTime=inf  FramePeriod=inf  OutMin=[]  OutMax=[]  OutDataTypeStr=Inherit: Inherit from 'Constant value'
  MC_Constant3 : lib2011b/Simulink Original/Sources/MC_Constant  Value=KACC_ACCUT_SW  datatype=Inherit: Inherit from 'Constant value'  SampleTime=inf  FramePeriod=inf  OutMin=[]  OutMax=[]  OutDataTypeStr=Inherit: Inherit from 'Constant value'
  MC_DataTypeConversion : lib2011b/Simulink Original/Signal Attributes/MC_DataTypeConversion  OutMin=[]  OutMax=[]  OutDataTypeStr=boolean  Signaltype=boolean  ConvertRealWorld=Real World Value (RWV)  RndMeth=Zero  SaturateOnIntegerOverflow=on  SampleTime=-1
  MC_LogicalOperator : lib2011b/Simulink Original/Logic and Bit Operations/MC_LogicalOperator  SelectedOperator=OR  Inputs=3  SampleTime=-1  AllPortsSameDT=off  OutDataTypeStr=boolean
  MC_LogicalOperator1 : lib2011b/Simulink Original/Logic and Bit Operations/MC_LogicalOperator  SelectedOperator=AND  Inputs=2  SampleTime=-1  AllPortsSameDT=off  OutDataTypeStr=boolean
  MC_LogicalOperator2 : lib2011b/Simulink Original/Logic and Bit Operations/MC_LogicalOperator  SelectedOperator=AND  Inputs=2  SampleTime=-1  AllPortsSameDT=off  OutDataTypeStr=boolean
  MC_RelationalOperator : lib2011b/Simulink Original/Logic and Bit Operations/MC_RelationalOperator  Operator=<=  SampleTime=-1  InputSameDT=on  OutDataTypeStr=boolean
  MC_RelationalOperator1 : lib2011b/Simulink Original/Logic and Bit Operations/MC_RelationalOperator  Operator=>=  SampleTime=-1  InputSameDT=on  OutDataTypeStr=boolean
  MC_RelationalOperator2 : lib2011b/Simulink Original/Logic and Bit Operations/MC_RelationalOperator  Operator=<=  SampleTime=-1  InputSameDT=on  OutDataTypeStr=boolean
  MC_Switch : lib2011b/Simulink Original/Signal Routing/MC_Switch  Criteria=u2 ~= 0  Threshold=0  SampleTime=-1  InputSameDT=on  OutMin=[]  OutMax=[]  AllowDiffInputSizes=off
  xis_colof : Outport
  wires:
  MC_RelationalOperator/1 -> MC_LogicalOperator1/1
  xirmd_iss/1 -> MC_LogicalOperator/3
  xismd_iss/1 -> MC_LogicalOperator/2
  vspe/1 -> MC_RelationalOperator/1
  MC_Constant/1 -> MC_RelationalOperator/2
  xstbymd_iss/1 -> MC_LogicalOperator1/2
  MC_LogicalOperator1/1 -> MC_LogicalOperator/1
  iss_state/1 -> MC_RelationalOperator1/1, MC_RelationalOperator2/1
  MC_Constant1/1 -> MC_RelationalOperator1/2
  MC_Constant2/1 -> MC_RelationalOperator2/2
  MC_RelationalOperator1/1 -> MC_LogicalOperator2/1
  MC_RelationalOperator2/1 -> MC_LogicalOperator2/2
  MC_Constant3/1 -> MC_DataTypeConversion/1
  MC_LogicalOperator2/1 -> MC_Switch/1
  MC_DataTypeConversion/1 -> MC_Switch/2
  MC_LogicalOperator/1 -> MC_Switch/3
  MC_Switch/1 -> xis_colof/1  "xis_colof"

== system filecuaho/acc_xaccuton/acc_accutreq/do_xlacfs ==
  xbrst : Inport
  xzst : Inport  Port=2
  xirmd_iss : Inport  Port=3
  LogicalOperator1 : lib2011b/Simulink Original/Logic and Bit Operations/MC_LogicalOperator  SelectedOperator=AND  Inputs=2  SampleTime=-1  AllPortsSameDT=off  OutDataTypeStr=boolean
  LogicalOperator2 : lib2011b/Simulink Original/Logic and Bit Operations/MC_LogicalOperator  SelectedOperator=AND  Inputs=2  SampleTime=-1  AllPortsSameDT=off  OutDataTypeStr=boolean
  LogicalOperator55 : lib2011b/Simulink Original/Logic and Bit Operations/MC_LogicalOperator  SelectedOperator=OR  Inputs=2  SampleTime=-1  AllPortsSameDT=off  OutDataTypeStr=boolean
  MC_LogicalOperator1 : lib2011b/Simulink Original/Logic and Bit Operations/MC_LogicalOperator  SelectedOperator=NOT  Inputs=2  SampleTime=-1  AllPortsSameDT=off  OutDataTypeStr=boolean
  xlacfs : Outport
  xlacfs_iss : Outport  Port=2
  wires:
  xzst/1 -> LogicalOperator55/2
  xbrst/1 -> LogicalOperator55/1
  LogicalOperator55/1 -> LogicalOperator1/1, LogicalOperator2/1
  xirmd_iss/1 -> LogicalOperator2/2, MC_LogicalOperator1/1
  MC_LogicalOperator1/1 -> LogicalOperator1/2
  LogicalOperator1/1 -> xlacfs/1  "xlacfs"
  LogicalOperator2/1 -> xlacfs_iss/1  "xlacfs_iss"

== system filecuaho/acc_xaccuton/acc_accutreq/do_xlacni ==
  ne : Inport
  Constant1 : lib2011b/Simulink Original/Sources/MC_Constant  Value=KSNACIH  datatype=Inherit: Inherit from 'Constant value'  SampleTime=inf  FramePeriod=inf  OutMin=[]  OutMax=[]  OutDataTypeStr=Inherit: Inherit from 'Constant value'
  Constant7 : lib2011b/Simulink Original/Sources/MC_Constant  Value=KSNACIH_HYS  datatype=Inherit: Inherit from 'Constant value'  SampleTime=inf  FramePeriod=inf  OutMin=[]  OutMax=[]  OutDataTypeStr=Inherit: Inherit from 'Constant value'
  MC_Hysteresis2 : SUBSYSTEM_LIB_CNV/TrueHys
      settings: AttributesFormatString=True
  xlacni : Outport
  wires:
  ne/1 -> MC_Hysteresis2/1
  Constant7/1 -> MC_Hysteresis2/3
  Constant1/1 -> MC_Hysteresis2/2
  MC_Hysteresis2/1 -> xlacni/1  "xlacni"

== system filecuaho/variable_compressor_control/vcv_cut_req/vcvcut_req ==
  note: ATシフトチェンジ中フラグ
  ne_smooth : Inport
  tqe_mx : Inport  Port=2
  des_tqei : Inport  Port=3
  gearp : Inport  Port=4
  xsftflg : Inport  Port=5
  MC_Add : lib2011b/Simulink Original/Math Operations/MC_Add  Inputs=+-  CollapseDim=1  SampleTime=-1  InputSameDT=on  OutMin=[]  OutMax=[]  OutDataTypeStr=single
  MC_Constant5 : lib2011b/Simulink Original/Sources/MC_Constant  Value=KACC_VCVCUT_NE  datatype=Inherit: Inherit from 'Constant value'  SampleTime=inf  FramePeriod=inf  OutMin=[]  OutMax=[]  OutDataTypeStr=Inherit: Inherit from 'Constant value'
  MC_Constant6 : lib2011b/Simulink Original/Sources/MC_Constant  Value=KACC_VCVCUT_GR_HI  datatype=Inherit: Inherit from 'Constant value'  SampleTime=inf  FramePeriod=inf  OutMin=[]  OutMax=[]  OutDataTypeStr=Inherit: Inherit from 'Constant value'
  MC_Constant7 : lib2011b/Simulink Original/Sources/MC_Constant  Value=KACC_VCVCUT_GR_LO  datatype=Inherit: Inherit from 'Constant value'  SampleTime=inf  FramePeriod=inf  OutMin=[]  OutMax=[]  OutDataTypeStr=Inherit: Inherit from 'Constant value'
  MC_Constant8 : lib2011b/Simulink Original/Sources/MC_Constant  Value=KACC_VCVCUT_TQDIF  datatype=Inherit: Inherit from 'Constant value'  SampleTime=inf  FramePeriod=inf  OutMin=[]  OutMax=[]  OutDataTypeStr=Inherit: Inherit from 'Constant value'
  MC_Constant9 : lib2011b/Simulink Original/Sources/MC_Constant  Value=KACC_VCVCUT_DESTQ  datatype=Inherit: Inherit from 'Constant value'  SampleTime=inf  FramePeriod=inf  OutMin=[]  OutMax=[]  OutDataTypeStr=Inherit: Inherit from 'Constant value'
  MC_LogicalOperator : lib2011b/Simulink Original/Logic and Bit Operations/MC_LogicalOperator  SelectedOperator=AND  Inputs=2  SampleTime=-1  AllPortsSameDT=off  OutDataTypeStr=boolean
  MC_LogicalOperator1 : lib2011b/Simulink Original/Logic and Bit Operations/MC_LogicalOperator  SelectedOperator=AND  Inputs=2  SampleTime=-1  AllPortsSameDT=off  OutDataTypeStr=boolean
  MC_LogicalOperator2 : lib2011b/Simulink Original/Logic and Bit Operations/MC_LogicalOperator  SelectedOperator=AND  Inputs=3  SampleTime=-1  AllPortsSameDT=off  OutDataTypeStr=boolean
  MC_LogicalOperator3 : lib2011b/Simulink Original/Logic and Bit Operations/MC_LogicalOperator  SelectedOperator=AND  Inputs=2  SampleTime=-1  AllPortsSameDT=off  OutDataTypeStr=boolean
  MC_LogicalOperator4 : lib2011b/Simulink Original/Logic and Bit Operations/MC_LogicalOperator  SelectedOperator=NOT  Inputs=2  SampleTime=-1  AllPortsSameDT=off  OutDataTypeStr=boolean
  MC_RelationalOperator : lib2011b/Simulink Original/Logic and Bit Operations/MC_RelationalOperator  Operator=>  SampleTime=-1  InputSameDT=on  OutDataTypeStr=boolean
  MC_RelationalOperator1 : lib2011b/Simulink Original/Logic and Bit Operations/MC_RelationalOperator  Operator=<=  SampleTime=-1  InputSameDT=on  OutDataTypeStr=boolean
  MC_RelationalOperator2 : lib2011b/Simulink Original/Logic and Bit Operations/MC_RelationalOperator  Operator=>=  SampleTime=-1  InputSameDT=on  OutDataTypeStr=boolean
  MC_RelationalOperator3 : lib2011b/Simulink Original/Logic and Bit Operations/MC_RelationalOperator  Operator=<  SampleTime=-1  InputSameDT=on  OutDataTypeStr=boolean
  MC_RelationalOperator4 : lib2011b/Simulink Original/Logic and Bit Operations/MC_RelationalOperator  Operator=>  SampleTime=-1  InputSameDT=on  OutDataTypeStr=boolean
  xvcv_cut_rq : Outport
  wires:
  ne_smooth/1 -> MC_RelationalOperator/1
  tqe_mx/1 -> MC_Add/1
  MC_LogicalOperator4/1 -> MC_LogicalOperator3/2
  xsftflg/1 -> MC_LogicalOperator4/1
  MC_LogicalOperator2/1 -> MC_LogicalOperator3/1
  MC_LogicalOperator1/1 -> MC_LogicalOperator2/2
  MC_LogicalOperator/1 -> MC_LogicalOperator2/3
  MC_RelationalOperator/1 -> MC_LogicalOperator2/1
  MC_RelationalOperator4/1 -> MC_LogicalOperator1/2
  MC_RelationalOperator3/1 -> MC_LogicalOperator1/1
  MC_Constant9/1 -> MC_RelationalOperator4/2
  MC_Constant8/1 -> MC_RelationalOperator3/2
  MC_Add/1 -> MC_RelationalOperator3/1
  des_tqei/1 -> MC_Add/2, MC_RelationalOperator4/1
  MC_RelationalOperator2/1 -> MC_LogicalOperator/2
  MC_RelationalOperator1/1 -> MC_LogicalOperator/1
  MC_Constant7/1 -> MC_RelationalOperator2/2
  gearp/1 -> MC_RelationalOperator1/1, MC_RelationalOperator2/1
  MC_Constant6/1 -> MC_RelationalOperator1/2
  MC_Constant5/1 -> MC_RelationalOperator/2
  MC_LogicalOperator3/1 -> xvcv_cut_rq/1  "xvcv_cut_rq"

== system filecuaho/acc_xaccuton/acc_accutreq/do_xacpcut/xcolphi ==
  colp : Inport
  Constant5 : lib2011b/Simulink Original/Sources/MC_Constant  Value=KACC_HIPS_ACON  datatype=Inherit: Inherit from 'Constant value'  SampleTime=inf  FramePeriod=inf  OutMin=[]  OutMax=[]  OutDataTypeStr=Inherit: Inherit from 'Constant value'
  Constant59 : lib2011b/Simulink Original/Sources/MC_Constant  Value=KACC_HIPS_ACOF  datatype=Inherit: Inherit from 'Constant value'  SampleTime=inf  FramePeriod=inf  OutMin=[]  OutMax=[]  OutDataTypeStr=Inherit: Inherit from 'Constant value'
  MC_Add : lib2011b/Simulink Original/Math Operations/MC_Add  Inputs=+-  CollapseDim=1  SampleTime=-1  InputSameDT=on  OutMin=[]  OutMax=[]  OutDataTypeStr=single
  MC_Hysteresis : SUBSYSTEM_LIB_CNV/TrueHys
      settings: AttributesFormatString=True
  xcolphi : Outport
  wires:
  MC_Hysteresis/1 -> xcolphi/1  "xcolphi"
  colp/1 -> MC_Hysteresis/1
  Constant59/1 -> MC_Hysteresis/2, MC_Add/1
  MC_Add/1 -> MC_Hysteresis/3
  Constant5/1 -> MC_Add/2

== system filecuaho/acc_xaccuton/acc_accutreq/do_xacpcut/xcolplo ==
  colp : Inport
  w_tsmpl : Inport  Port=2
  Constant1 : lib2011b/Simulink Original/Sources/MC_Constant  Value=0  datatype=single  SampleTime=inf  FramePeriod=inf  OutMin=[]  OutMax=[]  OutDataTypeStr=single
  Constant2 : lib2011b/Simulink Original/Sources/MC_Constant  Value=0  datatype=single  SampleTime=inf  FramePeriod=inf  OutMin=[]  OutMax=[]  OutDataTypeStr=single
  Constant3 : lib2011b/Simulink Original/Sources/MC_Constant  Value=KACC_COLPD  datatype=Inherit: Inherit from 'Constant value'  SampleTime=inf  FramePeriod=inf  OutMin=[]  OutMax=[]  OutDataTypeStr=Inherit: Inherit from 'Constant value'
  Constant4 : lib2011b/Simulink Original/Sources/MC_Constant  Value=false  datatype=Inherit: Inherit from 'Constant value'  SampleTime=inf  FramePeriod=inf  OutMin=[]  OutMax=[]  OutDataTypeStr=Inherit: Inherit from 'Constant value'
  Constant5 : lib2011b/Simulink Original/Sources/MC_Constant  Value=KACC_LOPS_ACON  datatype=Inherit: Inherit from 'Constant value'  SampleTime=inf  FramePeriod=inf  OutMin=[]  OutMax=[]  OutDataTypeStr=Inherit: Inherit from 'Constant value'
  Constant59 : lib2011b/Simulink Original/Sources/MC_Constant  Value=KACC_LOPS_ACOF  datatype=Inherit: Inherit from 'Constant value'  SampleTime=inf  FramePeriod=inf  OutMin=[]  OutMax=[]  OutDataTypeStr=Inherit: Inherit from 'Constant value'
  MC_Constant : lib2011b/Simulink Original/Sources/MC_Constant  Value=KCOLPLOTIME  datatype=Inherit: Inherit from 'Constant value'  SampleTime=inf  FramePeriod=inf  OutMin=[]  OutMax=[]  OutDataTypeStr=Inherit: Inherit from 'Constant value'
  MC_DownCounter : lib2011b/Mazda Library/Counter/MC_DownCounter  EnblRst=off
      settings: AttributesFormatString=Down Counter
  MC_DownCounter1 : lib2011b/Mazda Library/Counter/MC_DownCounter  EnblRst=off
      settings: AttributesFormatString=Down Counter
  MC_LogicalOperator1 : lib2011b/Simulink Original/Logic and Bit Operations/MC_LogicalOperator  SelectedOperator=NOT  Inputs=2  SampleTime=-1  AllPortsSameDT=off  OutDataTypeStr=boolean
  MC_LogicalOperator2 : lib2011b/Simulink Original/Logic and Bit Operations/MC_LogicalOperator  SelectedOperator=NOT  Inputs=2  SampleTime=-1  AllPortsSameDT=off  OutDataTypeStr=boolean
  MC_LowPass : lib2011b/Mazda Library/Filter/MC_LowPass
      settings: AttributesFormatString=LowPass
  MC_Product : lib2011b/Simulink Original/Math Operations/MC_Product  Inputs=*/  Multiplication=Element-wise(.*)  CollapseDim=1  SampleTime=-1  OutMin=[]  OutMax=[]  OutDataTypeStr=single  RndMeth=Zero
  MC_RelationalOperator : lib2011b/Simulink Original/Logic and Bit Operations/MC_RelationalOperator  Operator=<=  SampleTime=-1  InputSameDT=on  OutDataTypeStr=boolean
  MC_RelationalOperator1 : lib2011b/Simulink Original/Logic and Bit Operations/MC_RelationalOperator  Operator=>=  SampleTime=-1  InputSameDT=on  OutDataTypeStr=boolean
  MC_RelationalOperator2 : lib2011b/Simulink Original/Logic and Bit Operations/MC_RelationalOperator  Operator=<=  SampleTime=-1  InputSameDT=on  OutDataTypeStr=boolean
  MC_RelationalOperator3 : lib2011b/Simulink Original/Logic and Bit Operations/MC_RelationalOperator  Operator=<=  SampleTime=-1  InputSameDT=on  OutDataTypeStr=boolean
  MC_SetFlag : lib2011b/Mazda Library/Other/MC_SetFlag
      settings: AttributesFormatString=SetFlag
  xcolplo : Outport
  wires:
  Constant5/1 -> MC_RelationalOperator1/2
  Constant59/1 -> MC_RelationalOperator/2
  Constant4/1 -> MC_LowPass/3
  Constant3/1 -> MC_LowPass/2
  colp/1 -> MC_LowPass/1
  MC_LowPass/1 -> MC_RelationalOperator/1, MC_RelationalOperator1/1  "colpd"
  MC_Product/1 -> [w_colplo_init]  "w_colplo_init"
  [w_colplo_init] -> MC_DownCounter1/3
  [w_colplo_init] -> MC_DownCounter/3
  w_tsmpl/1 -> MC_Product/2
  MC_Constant/1 -> MC_Product/1
  MC_SetFlag/1 -> xcolplo/1  "xcolplo"
  MC_RelationalOperator3/1 -> MC_SetFlag/2
  MC_RelationalOperator2/1 -> MC_SetFlag/1
  Constant2/1 -> MC_RelationalOperator3/2
  Constant1/1 -> MC_RelationalOperator2/2
  MC_DownCounter/1 -> MC_RelationalOperator3/1  "ccolploset"
  MC_DownCounter1/1 -> MC_RelationalOperator2/1  "ccolplorst"
  MC_LogicalOperator2/1 -> MC_DownCounter/1
  MC_LogicalOperator1/1 -> MC_DownCounter1/1
  MC_RelationalOperator1/1 -> MC_LogicalOperator1/1, MC_DownCounter1/2
  MC_RelationalOperator/1 -> MC_LogicalOperator2/1, MC_DownCounter/2
